simulink model "System7b"  (R2021a)
settings: Solver=VariableStepAuto  StartTime=0.0  StopTime=10.0  RelTol=1e-3
values from neighbouring files (symbols this model uses):
  K1 = -2.2559    [Lab1_b_simulink.m]
  Kp = -20    [Lab1_b_simulink.m]
  tau_s = 0.0231    [Lab1_b_simulink.m]
settings Model: Creator=lucil  LastModifiedBy=lucil

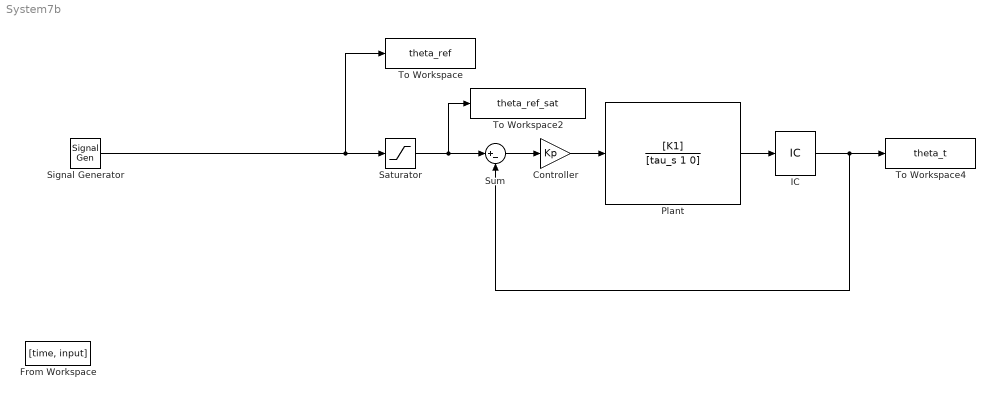
== system System7b ==
  Controller : Gain  Gain=Kp
  From Workspace : FromWorkspace  VariableName=[time, input]  SampleTime=0.001
  IC : InitialCondition  Value=-0.1
  Plant : TransferFcn  Numerator=[K1]  Denominator=[tau_s 1 0]
  Saturator : Saturate  UpperLimit=0.7  LowerLimit=-0.7
  Signal Generator : SignalGenerator  WaveForm=square  Frequency=0.4
  Sum : Sum  Inputs=|+-
  To Workspace : ToWorkspace  VariableName=theta_ref  SaveFormat=Timeseries  SampleTime=-1
  To Workspace2 : ToWorkspace  VariableName=theta_ref_sat  SaveFormat=Timeseries  SampleTime=-1
  To Workspace4 : ToWorkspace  VariableName=theta_t  SaveFormat=Timeseries  SampleTime=0.001
  wires:
  Controller/1 -> Plant/1
  Sum/1 -> Controller/1
  IC/1 -> To Workspace4/1, Sum/2
  Saturator/1 -> To Workspace2/1, Sum/1
  Signal Generator/1 -> To Workspace/1, Saturator/1
  Plant/1 -> IC/1
